simulink model "Project3_Trial"  (R2023b)
settings: Solver=VariableStepAuto  StartTime=0.0  StopTime=10.0  RelTol=1e-3
values from neighbouring files (symbols this model uses):
  b = 0.1    [Project3_Run_Trial.m]
  F = 1    [Project3_Run_Trial.m]
  k = 20    [Project3_Run_Trial.m]
  M = 1    [Project3_Run_Trial.m]
settings Model: Creator=mfb36  LastModifiedBy=mfb36

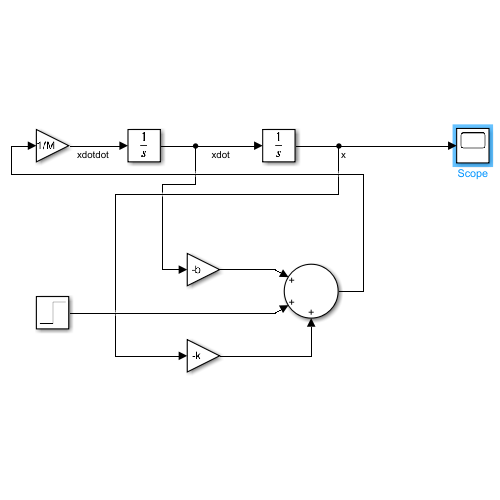
[thumbnail: Simulink's stored preview of the top-level diagram]
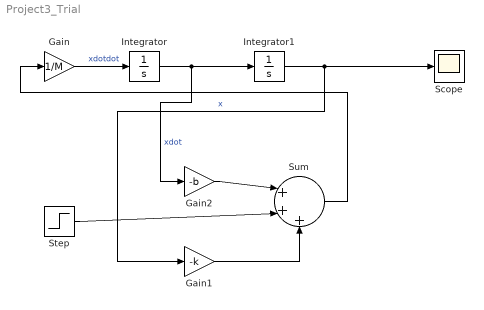
== system Project3_Trial ==
  Gain : Gain  Gain=1/M
  Gain1 : Gain  Gain=-k
  Gain2 : Gain  Gain=-b
  Integrator : Integrator
  Integrator1 : Integrator
  Scope : Scope
  Step : Step  After=F  SampleTime=0
  Sum : Sum  Inputs=|+++
  wires:
  Gain/1 -> Integrator/1  "xdotdot"
  Integrator/1 -> Gain2/1, Integrator1/1  "xdot"
  Integrator1/1 -> Scope/1, Gain1/1  "x"
  Gain2/1 -> Sum/1
  Gain1/1 -> Sum/3
  Step/1 -> Sum/2
  Sum/1 -> Gain/1
